simulink model "mcb_pmsm_foc_hall_f28069m_Hall_Sensor"  (R2022b)
settings: Solver=FixedStepDiscrete  StartTime=0.0  StopTime=8  RelTol=1e-3  EnableMultiTasking=on
InitFcn:
  | mcb_pmsm_foc_hall_f28069m_data;
undefined symbols (not defined in the file): Down, GPTRIP1SEL, GPTRIP2SEL, inverter, PI_params, pmsm, target, Ts, Ts_motor, Ts_simulink, Ts_speed, TZ1, TZ2, Up
libraries: simulink x14, mcbcontrolslib x9, mcbpositiondecoderlib x7, idelinklib_common x6, c2802xlib x5, c280xlib x5, slpidlib x3, c2806xlib x3, svdutilitieslib x2, c2000lib x1, mcbplantlib x1, autolibpmsmexterior x1
(part 3 of 3)

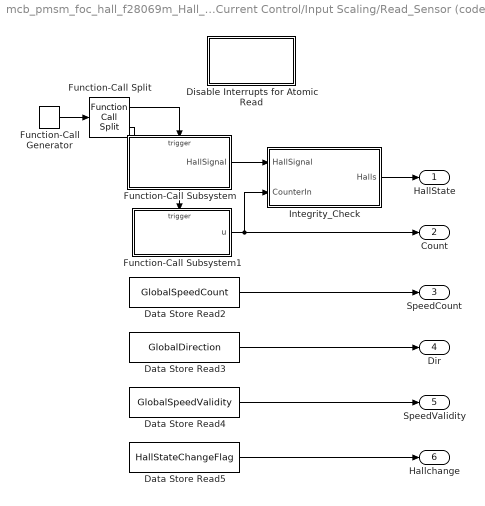
== system mcb_pmsm_foc_hall_f28069m_Hall_Sensor/Current Control/Input Scaling/Read_Sensor (codegen)/Calculate Position from Hall/Atomic Hall Reading ==
  Data Store Read2 : DataStoreRead  DataStoreName=GlobalSpeedCount  IndexOptions=Index vector (dialog)  Indices=1  OutputSizes=1
  Data Store Read3 : DataStoreRead  DataStoreName=GlobalDirection  IndexOptions=Index vector (dialog)  Indices=1  OutputSizes=1
  Data Store Read4 : DataStoreRead  DataStoreName=GlobalSpeedValidity  IndexOptions=Index vector (dialog)  Indices=1  OutputSizes=1
  Data Store Read5 : DataStoreRead  Priority=1  DataStoreName=HallStateChangeFlag  IndexOptions=Index vector (dialog)  Indices=1  OutputSizes=1
  Disable Interrupts for Atomic Read : Subsystem  mask(System Outputs){ShowInLibBrowser=0}
      mask prompts: ShowInLibBrowser "Simulink:masks:CustCodeMaskParam1_MP"
      settings: CopyFcn=cccopyfcn(gcb)  OpenFcn=ccopenfcn('System Outputs Function')
      mask Help: eval('feval(''rtwprivate'',''rtwhelpview'',''rtw_sys_outputs_block'')');
      mask Display: disp('System\nOutputs');
  Function-Call Generator : simulink/Ports & Subsystems/Function-Call Generator  sample_time=-1  numberOfIterations=1  DisallowWideOutput=off
  Function-Call Split : FunctionCallSplit  NumOutputPorts=2  OutputPortLayout=default
  Function-Call Subsystem : Subsystem  TreatAsAtomicUnit=on
  Function-Call Subsystem1 : Subsystem  TreatAsAtomicUnit=on
  Integrity_Check : Subsystem
  HallState : Outport
  Count : Outport  Port=2
  SpeedCount : Outport  Port=3
  Dir : Outport  Port=4
  SpeedValidity : Outport  Port=5
  Hallchange : Outport  Port=6
  wires:
  Data Store Read4/1 -> SpeedValidity/1
  Data Store Read5/1 -> Hallchange/1
  Data Store Read2/1 -> SpeedCount/1
  Data Store Read3/1 -> Dir/1
  Function-Call Split/1 -> Function-Call Subsystem/Trigger
  Integrity_Check/1(Halls) -> HallState/1
  Function-Call Split/2 -> Function-Call Subsystem1/Trigger
  Function-Call Generator/1 -> Function-Call Split/1
  Function-Call Subsystem/1(HallSignal) -> Integrity_Check/1(HallSignal)
  Function-Call Subsystem1/1(u) -> Count/1, Integrity_Check/2(CounterIn)

== system mcb_pmsm_foc_hall_f28069m_Hall_Sensor/Current Control/Input Scaling/Read_Sensor (codegen)/Calculate Position from Hall/Subsystem ==
  Input : Inport
  Enable : EnablePort
  Output : Outport
  wires:
  Input/1 -> Output/1

== system mcb_pmsm_foc_hall_f28069m_Hall_Sensor/Hardware Init/Code Generation/Calculate ADC Offset /For Iterator Subsystem/If Action Subsystem ==
  In1 : Inport
  In2 : Inport  Port=2
  Action Port : ActionPort  ActionPortLabel=if(u1 > 8)
  Memory : Memory  InheritSampleTime=on
  Memory1 : Memory  InheritSampleTime=on
  Sum : Sum
  Sum1 : Sum
  Out1 : Outport
  Out2 : Outport  Port=2
  wires:
  In1/1 -> Sum/1
  Sum/1 -> Out1/1, Memory/1
  In2/1 -> Sum1/1
  Memory/1 -> Sum/2
  Sum1/1 -> Out2/1, Memory1/1
  Memory1/1 -> Sum1/2

== system mcb_pmsm_foc_hall_f28069m_Hall_Sensor/Current Control/Input Scaling/Read_Sensor (codegen)/Calculate Position from Hall/Atomic Hall Reading/Disable Interrupts for Atomic Read ==

== system mcb_pmsm_foc_hall_f28069m_Hall_Sensor/Current Control/Input Scaling/Read_Sensor (codegen)/Calculate Position from Hall/Atomic Hall Reading/Function-Call Subsystem ==
  function : TriggerPort  TriggerType=function-call  VariantControl=Variant
  Bitwise AND : simulink/Logic and Bit Operations/Bitwise Operator  logicop=AND  UseBitMask=on  BitMask=hex2dec('07000000')  BitMaskRealWorld=Stored Integer
  Data Type Conversion : DataTypeConversion  OutDataTypeStr=uint32  ConvertRealWorld=Stored Integer (SI)  SaturateOnIntegerOverflow=off  RndMeth=Floor
  Memory Copy3 : svdutilitieslib/Memory Copy  copyFrom=Specified source code symbol  copyFromAddressSource=Specify via dialog  copyFromAddress=hex2dec('00001000')  copyFromSrcCode=&GpioDataRegs.GPADAT.all  dataTypeFrom=uint32  dataDimensionFrom=1  useOffsetFrom=off  offsetFromSrc=Specify via dialog  offsetFrom=0  strideFrom=1  copyTo=Output port  copyToAddressSource=Specify via dialog  copyToAddress=hex2dec('00002000')  copyToSrcCode=myVariableDst  dataTypeTo=uint32  useOffsetTo=off  offsetToSrc=Specify via dialog  offsetTo=0  strideTo=1  sampleTime=-1  useInitValue=off  initValueSrc=Specify constant value  initValue=1  initValueSrcCode=myInitValueVariable  useAsMask=off  maskOperator=bitwise AND  useTermValue=off  termValue=1  isRealtimeEnabled=off  emitCCBeforeWrite=off  CCBeforeWrite=/* Custom Code Before Write*/  emitCCAfterWrite=off  CCAfterWrite=/* Custom Code After Write*/  blockPlatform=arduinoert
  Shift Arithmetic : ArithShift  BitShiftNumber=24
  HallSignal : Outport
  wires:
  Data Type Conversion/1 -> HallSignal/1
  Shift Arithmetic/1 -> Data Type Conversion/1
  Bitwise AND/1 -> Shift Arithmetic/1
  Memory Copy3/1 -> Bitwise AND/1

== system mcb_pmsm_foc_hall_f28069m_Hall_Sensor/Current Control/Input Scaling/Read_Sensor (codegen)/Calculate Position from Hall/Atomic Hall Reading/Function-Call Subsystem1 ==
  function : TriggerPort  TriggerType=function-call  VariantControl=Variant
  Memory Copy : idelinklib_common/Memory Copy  copyFrom=Specified source code symbol  copyFromAddressSource=Specify via dialog  copyFromAddress=hex2dec('00001000')  copyFromSrcCode=&ECap1Regs.TSCTR  dataTypeFrom=uint32  dataDimensionFrom=1  useOffsetFrom=off  offsetFromSrc=Specify via dialog  offsetFrom=0  strideFrom=1  copyTo=Output port  copyToAddressSource=Specify via dialog  copyToAddress=hex2dec('00002000')  copyToSrcCode=myVariableDst  dataTypeTo=uint32  useOffsetTo=off  offsetToSrc=Specify via dialog  offsetTo=0  strideTo=1  sampleTime=-1  useInitValue=off  initValueSrc=Specify constant value  initValue=1  initValueSrcCode=myInitValueVariable  useAsMask=off  maskOperator=bitwise AND  useTermValue=off  termValue=1  isRealtimeEnabled=off  emitCCBeforeWrite=off  CCBeforeWrite=/* Custom Code Before Write*/  emitCCAfterWrite=off  CCAfterWrite=/* Custom Code After Write*/
  Memory Copy1 : idelinklib_common/Memory Copy  copyFrom=Specified source code symbol  copyFromAddressSource=Specify via dialog  copyFromAddress=hex2dec('00001000')  copyFromSrcCode=&ECap2Regs.TSCTR  dataTypeFrom=uint32  dataDimensionFrom=1  useOffsetFrom=off  offsetFromSrc=Specify via dialog  offsetFrom=0  strideFrom=1  copyTo=Output port  copyToAddressSource=Specify via dialog  copyToAddress=hex2dec('00002000')  copyToSrcCode=myVariableDst  dataTypeTo=uint32  useOffsetTo=off  offsetToSrc=Specify via dialog  offsetTo=0  strideTo=1  sampleTime=-1  useInitValue=off  initValueSrc=Specify constant value  initValue=1  initValueSrcCode=myInitValueVariable  useAsMask=off  maskOperator=bitwise AND  useTermValue=off  termValue=1  isRealtimeEnabled=off  emitCCBeforeWrite=off  CCBeforeWrite=/* Custom Code Before Write*/  emitCCAfterWrite=off  CCAfterWrite=/* Custom Code After Write*/
  Memory Copy2 : idelinklib_common/Memory Copy  copyFrom=Specified source code symbol  copyFromAddressSource=Specify via dialog  copyFromAddress=hex2dec('00001000')  copyFromSrcCode=&ECap3Regs.TSCTR  dataTypeFrom=uint32  dataDimensionFrom=1  useOffsetFrom=off  offsetFromSrc=Specify via dialog  offsetFrom=0  strideFrom=1  copyTo=Output port  copyToAddressSource=Specify via dialog  copyToAddress=hex2dec('00002000')  copyToSrcCode=myVariableDst  dataTypeTo=uint32  useOffsetTo=off  offsetToSrc=Specify via dialog  offsetTo=0  strideTo=1  sampleTime=-1  useInitValue=off  initValueSrc=Specify constant value  initValue=1  initValueSrcCode=myInitValueVariable  useAsMask=off  maskOperator=bitwise AND  useTermValue=off  termValue=1  isRealtimeEnabled=off  emitCCBeforeWrite=off  CCBeforeWrite=/* Custom Code Before Write*/  emitCCAfterWrite=off  CCAfterWrite=/* Custom Code After Write*/
  Min : MinMax  Inputs=3
  u : Outport
  wires:
  Memory Copy1/1 -> Min/2
  Memory Copy/1 -> Min/1
  Memory Copy2/1 -> Min/3
  Min/1 -> u/1

== system mcb_pmsm_foc_hall_f28069m_Hall_Sensor/Current Control/Input Scaling/Read_Sensor (codegen)/Calculate Position from Hall/Atomic Hall Reading/Integrity_Check ==
  HallSignal : Inport
  CounterIn : Inport  Port=2
  Compare To Constant : simulink/Logic and Bit Operations/Compare To Constant  relop=<  const=Ts*target.CPU_frequency*0.5  OutDataTypeStr=uint8
  If : If  IfExpression=u1 == 0
  Merge : Merge
  NOT : Logic  IconShape=distinctive  AllPortsSameDT=off  OutDataTypeStr=boolean
  No_Integrity_issue : Subsystem  TreatAsAtomicUnit=on
  Refresh_Halls : Subsystem  TreatAsAtomicUnit=on
  Relational Operator : RelationalOperator  Operator===  OutDataTypeStr=boolean  RndMeth=Simplest  InputSameDT=off
  Unit Delay : UnitDelay  SampleTime=-1  HasFrameUpgradeWarning=on
  Halls : Outport
  wires:
  Refresh_Halls/1(Out1) -> Merge/2
  HallSignal/1 -> Relational Operator/1, No_Integrity_issue/1(Counter), Unit Delay/1
  If/2 -> Refresh_Halls/Action
  Merge/1 -> Halls/1
  No_Integrity_issue/1(Out1) -> Merge/1
  If/1 -> No_Integrity_issue/Action
  CounterIn/1 -> Compare To Constant/1
  Compare To Constant/1 -> NOT/2
  Relational Operator/1 -> NOT/1
  NOT/1 -> If/1
  Unit Delay/1 -> Relational Operator/2

== system mcb_pmsm_foc_hall_f28069m_Hall_Sensor/Current Control/Input Scaling/Read_Sensor (codegen)/Calculate Position from Hall/Atomic Hall Reading/Integrity_Check/No_Integrity_issue ==
  Counter : Inport
  Action Port : ActionPort
  Out1 : Outport
  wires:
  Counter/1 -> Out1/1

== system mcb_pmsm_foc_hall_f28069m_Hall_Sensor/Current Control/Input Scaling/Read_Sensor (codegen)/Calculate Position from Hall/Atomic Hall Reading/Integrity_Check/Refresh_Halls ==
  Action Port : ActionPort
  Bitwise AND : simulink/Logic and Bit Operations/Bitwise Operator  logicop=AND  UseBitMask=on  BitMask=hex2dec('07000000')  BitMaskRealWorld=Stored Integer
  Data Type Conversion : DataTypeConversion  OutDataTypeStr=uint32  ConvertRealWorld=Stored Integer (SI)  SaturateOnIntegerOverflow=off  RndMeth=Floor
  Memory Copy3 : svdutilitieslib/Memory Copy  copyFrom=Specified source code symbol  copyFromAddressSource=Specify via dialog  copyFromAddress=hex2dec('00001000')  copyFromSrcCode=&GpioDataRegs.GPADAT.all  dataTypeFrom=uint32  dataDimensionFrom=1  useOffsetFrom=off  offsetFromSrc=Specify via dialog  offsetFrom=0  strideFrom=1  copyTo=Output port  copyToAddressSource=Specify via dialog  copyToAddress=hex2dec('00002000')  copyToSrcCode=myVariableDst  dataTypeTo=uint32  useOffsetTo=off  offsetToSrc=Specify via dialog  offsetTo=0  strideTo=1  sampleTime=-1  useInitValue=off  initValueSrc=Specify constant value  initValue=1  initValueSrcCode=myInitValueVariable  useAsMask=off  maskOperator=bitwise AND  useTermValue=off  termValue=1  isRealtimeEnabled=off  emitCCBeforeWrite=off  CCBeforeWrite=/* Custom Code Before Write*/  emitCCAfterWrite=off  CCAfterWrite=/* Custom Code After Write*/  blockPlatform=arduinoert
  Shift Arithmetic : ArithShift  BitShiftNumber=24
  Out1 : Outport
  wires:
  Memory Copy3/1 -> Bitwise AND/1
  Bitwise AND/1 -> Shift Arithmetic/1
  Shift Arithmetic/1 -> Data Type Conversion/1
  Data Type Conversion/1 -> Out1/1

== matlab function mcb_pmsm_foc_hall_f28069m_Hall_Sensor/Current Control/Control_System/Current_Controllers/MATLAB Function ==
  data: dref input; dsat output; qref input; qsat output; saturation_mode input; saturation_limit input
function [dsat, qsat] = dqlimiter_custom(dref,qref, saturation_mode, saturation_limit)

switch saturation_mode

    case 0 % DQ Equivalentes
    mag=sqrt(dref^2 +qref^2);

    if(mag>saturation_limit)
        dsat=dref*saturation_limit/mag;
        qsat=qref*saturation_limit/mag;
    else
        dsat=dref;
        qsat=qref;
    end
    
    case 1 %Priorizado D
        %Establece el valor d al máximo de la saturacion (tanto en negativo
        %como en positivo)
        dsat=min(max(dref,-saturation_limit),saturation_limit);

        %Funcion sign devuelve el signo. Utiliza el limite de saturacion
        %restante para la q. Si d ya es limite, no hay q
        qsat=sign(qref)*min(abs(qref),sqrt(abs(saturation_limit^2-dsat^2)));

    case 2%Priorizado Q
        qsat=min(max(qref,-saturation_limit),saturation_limit);
        dsat=sign(dref)*min(abs(dref),sqrt(abs(saturation_limit^2-qsat^2)));

    otherwise%Error en la selecion, No deberia darse nunca
        qsat=qref;
        dsat=dref;

end

== matlab function mcb_pmsm_foc_hall_f28069m_Hall_Sensor/Inverter and Motor - Plant Model/Simulation/Sensor_Measurements/MATLAB Function ==
  data: pos_abs input; pos_rel output; paso input
function pos_rel = mod_custom(pos_abs, paso)
%Funcion floor devuelve la parte entera menor. 
pos_rel = pos_abs - paso*floor(pos_abs/paso);

== matlab function mcb_pmsm_foc_hall_f28069m_Hall_Sensor/Inverter and Motor - Plant Model/Simulation/Sensor_Measurements/MATLAB Function1 ==
  data: pos input; HA output; HB output; HC output
function [HA,HB,HC] = hallSimulator(pos)

%Habria que aplicar retrasos equivalentes al ancho de banda

pos=pos*360;

if(pos<90 | pos>270)
    HA=true;
else
    HA=false;
end
if(pos<210 & pos>30)
    HB=true;
else
    HB=false;
end

if(pos<330 & pos>150)
    HC=true;
else
    HC=false;
end

== matlab function mcb_pmsm_foc_hall_f28069m_Hall_Sensor/Inverter and Motor - Plant Model/Simulation/Sensor_Measurements/MATLAB Function2 ==
  data: HA input; sector output; HB input; HC input
function sector = HallASensor(HA,HB,HC)

%Error si es 0, todos los Halls estarian en el mismo polo
sector=0;
if(HA*~HB*HC==1)
    sector=5;
end
if(HA*~HB*~HC==1)
    sector=4;
end
if(HA*HB*~HC==1)
   sector=6;
end

if(~HA*HB*~HC==1)
    sector=2;
end
if(~HA*HB*HC==1)
    sector=3;
end
if(~HA*~HB*HC==1)
    sector=1;
end

== matlab function mcb_pmsm_foc_hall_f28069m_Hall_Sensor/Inverter and Motor - Plant Model/Simulation/Sensor_Measurements/MATLAB Function3 ==
  data: sector input; angulo_discreitzado output
function angulo_discreitzado = SectorAngulo(sector)

%Error si no estamos en algun sector
angulo_discreitzado=-1; 

    switch(sector)
        case 1
            angulo_discreitzado=240;
        case 2
            angulo_discreitzado=120;  
        case 3
            angulo_discreitzado=180;
        case 4
            angulo_discreitzado=0;
        case 5
            angulo_discreitzado=300;  
        case 6
            angulo_discreitzado=60;
    end

== matlab function mcb_pmsm_foc_hall_f28069m_Hall_Sensor/Inverter and Motor - Plant Model/Simulation/Sensor_Measurements/MATLAB Function4 ==
  data: sentido input; angulo_actual output; angulo_discretizado input; tiempo_actual input
function  angulo_actual= MedioAproximado(sentido,angulo_discretizado,tiempo_actual)

%Sentido 1 si es horario, -1 si es antihorario
angulo_discretizado=mod(angulo_discretizado+sentido*30,360);

% Angulo_anterior, tiempo_anterior y velocidad_anterior variables
% persistentes

persistent angulo_anterior
if isempty(angulo_anterior)
    angulo_anterior=180;
end
persistent tiempo_anterior
if isempty(tiempo_anterior)
    tiempo_anterior=-0.1;
end
persistent velocidad_anterior
if isempty(velocidad_anterior)
    velocidad_anterior=0; 
end

if(angulo_discretizado ~= angulo_anterior)
    velocidad_anterior=-1*sentido*60/(tiempo_actual-tiempo_anterior); 
    tiempo_anterior=tiempo_actual;
    angulo_anterior=angulo_discretizado;
end

angulo_actual=mod(angulo_discretizado+velocidad_anterior*(tiempo_actual-tiempo_anterior),360);

angulo_actual=angulo_actual/360;
